simulink model "ENGR490rover2DMoonOmega"  (R2023b)
settings: Solver=ode4  StartTime=0.0  StopTime=inf  FixedStep=0.1  RelTol=1e-3
model workspace (MAT data in the model file):
  vehicleTest = Simulink.Signal
  vehicleTest.DataType = 'Bus: VehicleTestBus'
  vehicleTest.Dimensions = -1
  vehicleTest.DimensionsMode = 'auto'
  vehicleTest.Complexity = 'auto'
  vehicleTest.SampleTime = -1
  vehicleTest.SamplingMode = 'auto'
  vehicleTest.InitialValue = 'vehicleTestInit'
values from neighbouring files (symbols this model uses):
  InitialState = [vehicleTest.init.pos vehicleTest.init.vel vehicleTest.init.phi vehicleTest.init.omega vehicleTest.init.charge vehicleTest.habitat.init.temp]    [ENGR490rover2DMoonOmegaParameters.m]
  vehicleTestInit = vehicleTest    [ENGR490rover2DMoonOmegaParameters.m]
libraries: simulink x2
settings Model: Creator=erau  LastModifiedBy=Alex
settings ModelReferenceCC: EnableRefExpFcnMdlSchedulingChecks=on

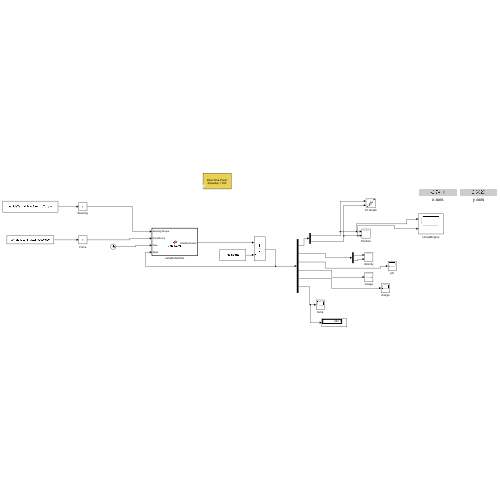
[thumbnail: Simulink's stored preview of the top-level diagram]
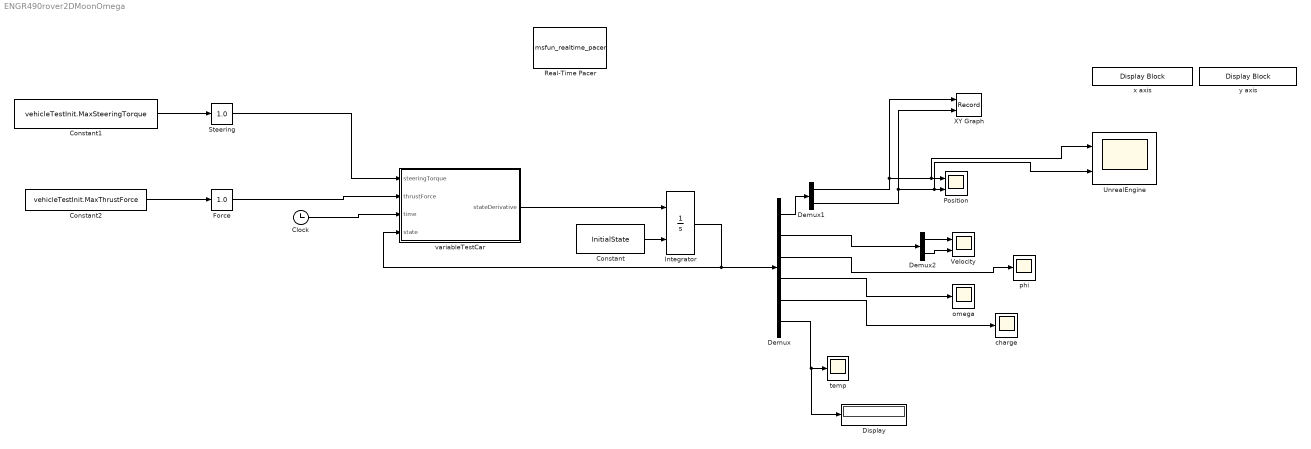
== system ENGR490rover2DMoonOmega ==
  Clock : Clock
  Constant : Constant  Value=InitialState  VectorParams1D=off
  Constant1 : Constant  Value=vehicleTestInit.MaxSteeringTorque
  Constant2 : Constant  Value=vehicleTestInit.MaxThrustForce
  Demux : Demux  Outputs=[2 2 1 1 1 1]
  Demux1 : Demux  Outputs=2
  Demux2 : Demux  Outputs=2
  Display : Display
  Force : simulink/Math Operations/Slider Gain  gain=1.0  low=-1  high=1
  Integrator : Integrator  InitialConditionSource=external
  Position : Scope  NumInputPorts=2
  Real-Time Pacer : M-S-Function  AncestorBlock=realtime_pacer_lib/Real-Time Pacer  FunctionName=msfun_realtime_pacer  Parameters=simTimePerRealTime  mask(RealTime_Pacer){simTimePerRealTime=300}
      mask prompts: simTimePerRealTime "Speedup (Simulation Time / Real Time):"
      mask help:
      | Slow down a simulation to track real (i.e., wall clock) elapsed time.
      |
      | "Speedup" specifies the ratio between simulation time and real time
      | • Speedup = N => N sec. of simulation time per sec. of real time
      | • Speedup can be fractional (e.g., 0.5, 1.3).
      | • Speedup = inf => allow simulation to run at full speed
      |
      | Click on the Help button for details.
      mask Help: web('realtime_pacer_help.html', '-helpbrowser')
      mask Display: fprintf('Real-Time Pacer\nSpeedup = %g', simTimePerRealTime)
  Steering : simulink/Math Operations/Slider Gain  gain=1.0  low=-1  high=1
  UnrealEngine : Scope  NumInputPorts=2
  Velocity : Scope  NumInputPorts=2
  XY Graph : Record  FileSettingsInternal="{\"entries\":[{\"content\":{\"excelSettings\":{\"content\":{},\"type\":\"Streamout.ExcelSettings\"}},\"type\":\"Streamout.FileSettingStorage\",\"uuid\":\"\"}],\"packageUris\":[\"http:\\/\\/schema.mathworks.com\\/mf0\\/streamout_blocks\\/R2020a\"],\"version\":\"1.0\"}"  Layout=[1 1]  SignalsInternal="{\"entries\":[{\"content\":{\"signals\":[{\"content\":{\"blockPath\":[],\"dimensions\":[1,1],\"domain\":\"\",\"lineColor\":\"#edb120\",\"plots\":[1],\"port\":1,\"sid\":[\"\"],\"signalID\":21,\"signalName\":\"Demux1:1\"},\"type\":\"RecordBlkView.Signal\",\"uuid\":\"\"},{\"content\":{\"blockPath\":[],\"dimensions\":[1,1],\"domain\":\"\",\"lineColor\":\"#7e2f8e\",\"plots\":[1],\"port\":2,\"sid\":[\"\"],\"signalID\":25,\"signalName\":\"Demux1:2\"},\"type\":\"RecordBlkView.Signal\",\"uuid\":\"\"}]},\"type\":\"RecordBlkView.InputSignals\",\"uuid\":\"\"}],\"packageUris\":[\"http:\\/\\/schema.mathworks.com\\/mf0\\/streamout_blocks\\/R2020a\"],\"version\":\"1.0\"}"  VisualizationBindings="{\"xyplotplugin\":{\"info\":[{\"series\":[{\"bindingParametersList\":[{\"parameter\":\"Y-Axis\",\"signalID\":25,\"signalName\":\"Demux1:2\"},{\"parameter\":\"X-Axis\",\"signalID\":21,\"signalName\":\"Demux1:1\"}],\"seriesID\":59742}],\"subplotID\":1}]}}"  CompatibilityTag=XY
  charge : Scope
  omega : Scope
  phi : Scope
  temp : Scope
  variableTestCar : MATLAB Function  TreatAsAtomicUnit=on
  x axis : DisplayBlock  LabelPosition=Hide  Transparency=1
  y axis : DisplayBlock  LabelPosition=Hide  Transparency=1
  wires:
  Clock/1 -> variableTestCar/3(time)
  variableTestCar/1(stateDerivative) -> Integrator/1
  Integrator/1 -> Demux/1, variableTestCar/4(state)
  Constant/1 -> Integrator/2
  Demux/1 -> Demux1/1
  Demux1/1 -> XY Graph/1, UnrealEngine/1, Position/1
  Demux1/2 -> XY Graph/2, UnrealEngine/2, Position/2
  Demux2/2 -> Velocity/2
  Demux2/1 -> Velocity/1
  Demux/2 -> Demux2/1
  Constant1/1 -> Steering/1
  Steering/1 -> variableTestCar/1(steeringTorque)
  Constant2/1 -> Force/1
  Force/1 -> variableTestCar/2(thrustForce)
  Demux/5 -> charge/1
  Demux/4 -> omega/1
  Demux/3 -> phi/1
  Demux/6 -> Display/1, temp/1

== matlab function ENGR490rover2DMoonOmega/variableTestCar ==
  settings: updateMethod=DISCRETE
  data: steeringTorque input; thrustForce input; time input; stateDerivative output; vehicleTest data_store_memory; state input
function stateDerivative = vehicleVar(steeringTorque, thrustForce, time,state)

%% Model of a vehicle in a plane
%  Input:      time and state: [rx ry vx vy phi charge]
%               
%  Output:     derivative of the state: [vx vy ax ay omega power]
%              
% 
%  Karl H. Siebold, February 2023
%  Embry Riddle Aeronautical University
%  Worldwide Campus

global vehicleTest

r      = state(1:2);        % [m]     position in x-y coordinates
v      = state(3:4);        % [m/s]   velocity in x-y coordinates
phi    = state(5);          % [rad]   heading
omega  = state(6);          % [rad/s] rate of the heading change
charge = state(7);          % [Ws]    charge of the battery
T   = state(8);          % [K]     temperature

%% Kinematics
vmag   = sqrt(v(1)^2 + v(2)^2);                            % magnitude of the velocity

Mpath2xy = [cos(phi) -sin(phi); sin(phi) cos(phi)];       % transformation from path ccordinates to x-y coordinates

adrag = vehicleTest.cd*v;                                 % drag as a linear function of the velocity, opposite the velocity vector

vdot      = thrustForce/vehicleTest.mass;

apath     =  [vdot; omega*vmag];                            % [m/s^2]  acceleration on the path coordinate system
a         =  Mpath2xy*apath - adrag';                       % [m/s^2]  transformed acceleration into the x-y coordinate system

omegaDot  = (steeringTorque - vehicleTest.SteeringDamping*omega)/vehicleTest.Inertia;      % [rad/s^2] Angular rate acceleration due to the steering torque and its damping

%% Power
power     = thrustForce*vmag;

%% Total heat balance
qConductionWidthWalls = sum(vehicleTest.habitat.width.wall.k.* vehicleTest.habitat.wall.width.area.*(vehicleTest.environment.moon.temperature - T));
qConductionLengthWalls = sum(vehicleTest.habitat.length.wall.k .* vehicleTest.habitat.wall.length.area .* (vehicleTest.environment.moon.temperature - T));
qConductionRoof = vehicleTest.habitat.roof.k * vehicleTest.habitat.roof.area * (vehicleTest.environment.moon.temperature - T);
qConductionFloor = vehicleTest.habitat.floor.k * vehicleTest.habitat.floor.area * (vehicleTest.environment.moon.temperature - T);

qRadiationWidthWalls = sum(vehicleTest.habitat.width.wall.eps .* vehicleTest.habitat.wall.width.area .* vehicleTest.environment.sigma .* ((vehicleTest.environment.moon.temperature)^4 - T^4));
qRadiationLengthWalls = sum(vehicleTest.habitat.length.wall.eps .* vehicleTest.habitat.wall.length.area .* vehicleTest.environment.sigma .* ((vehicleTest.environment.moon.temperature)^4 - T^4));
qRadiationRoof = vehicleTest.habitat.roof.eps * vehicleTest.habitat.roof.area * vehicleTest.environment.sigma * ((vehicleTest.environment.moon.temperature)^4 - T^4);

% Q_in = cross_sectional_area*(alphaVis*qSun+alphaIR*vehicleTest.environment.qEarth);
% qTotal = sum(vehicleTest.habitat.heat.qOut) + vehicleTest.habitat.roof.alph * qSun + qConductionWidthWalls+qConductionLengthWalls + qConductionRoof + qConductionFloor + qRadiationWidthWalls + qRadiationLengthWalls + qRadiationRoof;
% Q_out = 
%% Total specific heat times mass
cpmTotal = sum(vehicleTest.habitat.wall.cp .* vehicleTest.habitat.wall.mass) + vehicleTest.habitat.floor.cp * vehicleTest.habitat.floor.mass + vehicleTest.habitat.roof.cp * vehicleTest.habitat.roof.mass;

% use m*cp*dT/dt = Qin - Qout as first order differential equation, 
% i.e. model equation
tMod = mod(time, 100);  % 2548000
if tMod < 20
    % qSun    = 0.0;   % Night
    if T > 27+273.15
        qHeater =  0;
    else
        qHeater = sum(vehicleTest.habitat.heat.qOut);
    end
    % alphaVis=0.0;
    qTotal = qHeater-(qConductionWidthWalls+qConductionLengthWalls+qConductionRoof+qConductionFloor+qRadiationWidthWalls+qRadiationLengthWalls+qRadiationRoof);
else                 % Day
    % qSun = vehicleTest.environment.qSun;
    if T < 18+273.15
        qHeater = 30000;
        qAC = 0;
    else
        qHeater = 0;
        if T>27+273.15
            qAC = 1000;
        else
            qAC = 0;
        end
    end
    % alphaVis = vehicleTest.habitat.alphaVis;
    qTotal = qRadiationWidthWalls+qRadiationLengthWalls+qRadiationRoof+qConductionWidthWalls+qConductionLengthWalls+qConductionRoof+qConductionFloor+qHeater-qAC;
end

Tderiv = qTotal/cpmTotal;

%%%%%%%%%%%%%%%%%%%%%%%%%%%%%%%%%%%%%%%%%%%%%%
%% State Derivative
stateDerivative = [v(1) v(2) a(1) a(2) omega omegaDot -power Tderiv];                          % state derivative, velocity, acceleration, rotation, and charge

end
